simulink model "uas_sim"  (R2020b)
settings: Solver=VariableStepAuto  StartTime=0.0  StopTime=10.0  RelTol=1e-3  SampleTimeConstraint=STIndependent
undefined symbols (not defined in the file): Aircraft, datetime, datevec, Earth, Env, InitCond, WGS84
libraries: aerolibconvert2 x8, simulink x8, aerolibadyn x3, aerolibasang x3, aerolibtransform2 x2, aerolibatmos2 x1, sharedutil x1, aerolibbdyn x1, shared6dof x1, aerolibgravity2 x1
(part 1 of 2)
settings Model: Creator=brian  LastModifiedBy=brian

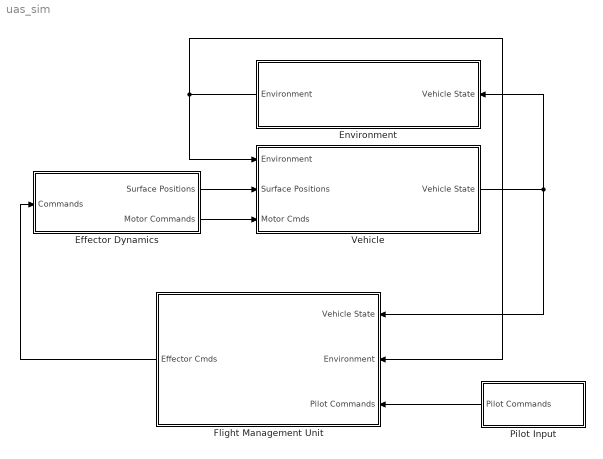
== system uas_sim ==
  Effector Dynamics : Subsystem
      settings: PortSchema="{\"entries\":[{\"content\":{\"sides\":[{\"content\":{\"connectorIds\":[]},\"type\":\"ConnectorPlacement.EquallySpacedRectSide\",\"uuid\":\"b20f7590-d69b-48b8-beb1-2fb7d3ab0357\"},{\"content\":{\"connectorIds\":[],\"side\":\"RIGHT\"},\"type\":\"ConnectorPlacement.EquallySpacedRectSide\",\"uuid\":\"07801f8a-7756-483e-a050-3c2fccc33404\"},{\"content\":{\"connectorIds\":[\"Out1\",\"Out2\"],\"side\":\"TOP\"},\"type\":\"ConnectorPlacement.EquallySpacedRectSide\",\"uuid\":\"ce3c3c94-ed36-4103-b079-69dcaeaf21e9\"},{\"content\":{\"connectorIds\":[\"In1\"],\"side\":\"BOTTOM\"},\"type\":\"ConnectorPlacement.EquallySpacedRectSide\",\"uuid\":\"ba78b819-a471-4bc3-b479-e6a973cfe14f\"},{\"content\":{\"connectorIds\":[],\"side\":\"HIDDEN\"},\"type\":\"ConnectorPlacement.EquallySpacedRectSide\",\"uuid\":\"3cf915a5-25a1-4380-9090-9561533312da\"}]},\"type\":\"ConnectorPlacement.EquallySpacedConnector\",\"uuid\":\"7ef4ddaa-ccd2-4778-89ce-8b4685524e82\"}],\"packageUris\":[\"http://schema.mathworks.com/mf0/Connector/R2020b\"],\"version\":\"1.0\"}"
  Environment : Subsystem
  Flight Management Unit : Subsystem
  Pilot Input : Subsystem
  Vehicle : Subsystem
  wires:
  Vehicle/1(Vehicle State) -> Environment/1(Vehicle State), Flight Management Unit/1(Vehicle State)
  Pilot Input/1(Pilot Commands) -> Flight Management Unit/3(Pilot Commands)
  Environment/1(Environment) -> Vehicle/1(Environment), Flight Management Unit/2(Environment)
  Flight Management Unit/1(Effector Cmds) -> Effector Dynamics/1(Commands)
  Effector Dynamics/1(Surface Positions) -> Vehicle/2(Surface Positions)
  Effector Dynamics/2(Motor Commands) -> Vehicle/3(Motor Cmds)

== system uas_sim/Effector Dynamics ==
  Commands : Inport
  Actuator Dynamics : Subsystem
  Bus Selector : BusSelector  OutputSignals=PWM,SBUS
  Mux : Mux  Inputs=2
  Selector : Selector  InputPortWidth=Aircraft.Eff.nCh  IndexOptions=Index vector (dialog)  Indices=Aircraft.Surf.map  OutputSizes=1
  Selector1 : Selector  InputPortWidth=Aircraft.Eff.nCh  IndexOptions=Index vector (dialog)  Indices=Aircraft.Motor.map  OutputSizes=1
  Surface Positions : Outport
  Motor Commands : Outport  Port=2
  wires:
  Commands/1 -> Bus Selector/1
  Bus Selector/1 -> Mux/1  "<PWM>"
  Bus Selector/2 -> Mux/2  "<SBUS>"
  Mux/1 -> Selector1/1, Selector/1
  Actuator Dynamics/1(Position) -> Surface Positions/1
  Selector/1 -> Actuator Dynamics/1(Command)
  Selector1/1 -> Motor Commands/1

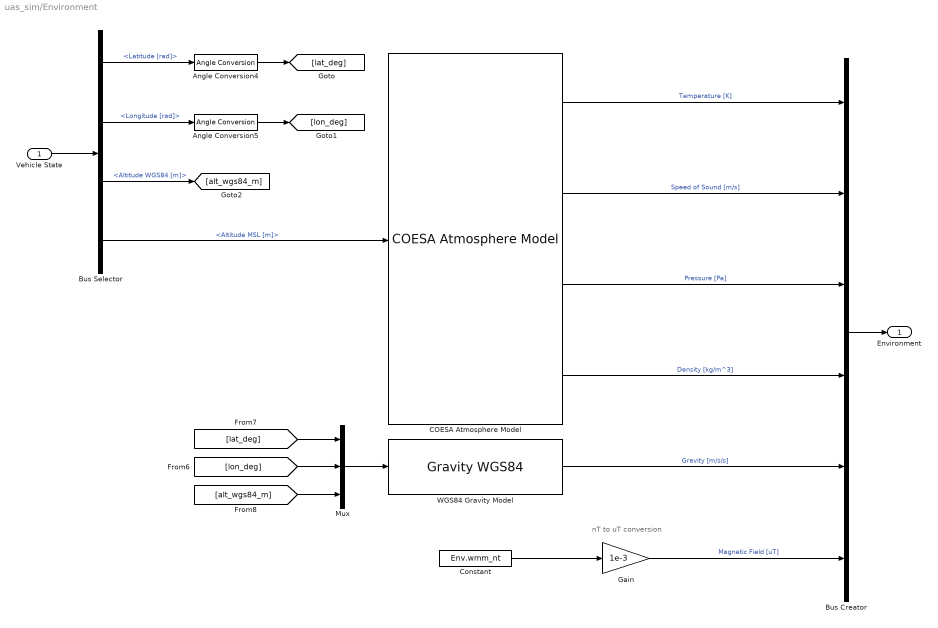
== system uas_sim/Environment ==
  note: nT to uT conversion
  Vehicle State : Inport
  Angle Conversion4 : aerolibconvert2/Angle Conversion  IU=rad  OU=deg
  Angle Conversion5 : aerolibconvert2/Angle Conversion  IU=rad  OU=deg
  Bus Creator : BusCreator  Inputs=6
  Bus Selector : BusSelector  OutputSignals=Latitude [rad],Longitude [rad],Altitude WGS84 [m],Altitude MSL [m]
  COESA Atmosphere Model : aerolibatmos2/COESA Atmosphere Model  units=Metric (MKS)  spec=1976 COESA-extended U.S. Standard Atmosphere  model=Profile  profile_var=High temperature  profile_percent=1%  profile_alt=5 km (16404 ft)  envelope_var=High temperature  envelope_percent=1%  action=Warning
  Constant : Constant  Value=Env.wmm_nt
  Gain : Gain  Gain=1e-3
  Mux : Mux  Inputs=3
  "WGS84 Gravity Model  " : GravityWGS84
  Environment : Outport
  wires:
  [lon_deg] -> Mux/2
  COESA Atmosphere Model/4 -> Bus Creator/4  "Density [kg/m^3]"
  Mux/1 -> "WGS84 Gravity Model  "/1
  Bus Selector/3 -> [alt_wgs84_m]  "<Altitude WGS84 [m]>"
  Vehicle State/1 -> Bus Selector/1
  Bus Selector/2 -> Angle Conversion5/1  "<Longitude [rad]>"
  COESA Atmosphere Model/2 -> Bus Creator/2  "Speed of Sound [m/s]"
  Bus Selector/4 -> COESA Atmosphere Model/1  "<Altitude MSL [m]>"
  [alt_wgs84_m] -> Mux/3
  Angle Conversion4/1 -> [lat_deg]
  [lat_deg] -> Mux/1
  Bus Creator/1 -> Environment/1
  Constant/1 -> Gain/1
  Gain/1 -> Bus Creator/6  "Magnetic Field [uT]"
  "WGS84 Gravity Model  "/1 -> Bus Creator/5  "Gravity [m/s/s]"
  Bus Selector/1 -> Angle Conversion4/1  "<Latitude [rad]>"
  COESA Atmosphere Model/3 -> Bus Creator/3  "Pressure [Pa]"
  COESA Atmosphere Model/1 -> Bus Creator/1  "Temperature [K]"
  Angle Conversion5/1 -> [lon_deg]

== system uas_sim/Flight Management Unit ==
  Vehicle State : Inport
  Environment : Inport  Port=2
  Pilot Commands : Inport  Port=3
  SenProc Model : Subsystem
      settings: PortSchema="{\"entries\":[{\"content\":{\"sides\":[{\"content\":{\"connectorIds\":[]},\"type\":\"ConnectorPlacement.EquallySpacedRectSide\",\"uuid\":\"b20f7590-d69b-48b8-beb1-2fb7d3ab0357\"},{\"content\":{\"connectorIds\":[],\"side\":\"RIGHT\"},\"type\":\"ConnectorPlacement.EquallySpacedRectSide\",\"uuid\":\"07801f8a-7756-483e-a050-3c2fccc33404\"},{\"content\":{\"connectorIds\":[\"In1\",\"In2\"],\"side\":\"TOP\"},\"type\":\"ConnectorPlacement.EquallySpacedRectSide\",\"uuid\":\"ce3c3c94-ed36-4103-b079-69dcaeaf21e9\"},{\"content\":{\"connectorIds\":[\"Out1\"],\"side\":\"BOTTOM\"},\"type\":\"ConnectorPlacement.EquallySpacedRectSide\",\"uuid\":\"ba78b819-a471-4bc3-b479-e6a973cfe14f\"},{\"content\":{\"connectorIds\":[],\"side\":\"HIDDEN\"},\"type\":\"ConnectorPlacement.EquallySpacedRectSide\",\"uuid\":\"3cf915a5-25a1-4380-9090-9561533312da\"}]},\"type\":\"ConnectorPlacement.EquallySpacedConnector\",\"uuid\":\"7ef4ddaa-ccd2-4778-89ce-8b4685524e82\"}],\"packageUris\":[\"http://schema.mathworks.com/mf0/Connector/R2020b\"],\"version\":\"1.0\"}"
  Sensor Models : Subsystem
      settings: PortSchema="{\"entries\":[{\"content\":{\"sides\":[{\"content\":{\"connectorIds\":[]},\"type\":\"ConnectorPlacement.EquallySpacedRectSide\",\"uuid\":\"b20f7590-d69b-48b8-beb1-2fb7d3ab0357\"},{\"content\":{\"connectorIds\":[],\"side\":\"RIGHT\"},\"type\":\"ConnectorPlacement.EquallySpacedRectSide\",\"uuid\":\"07801f8a-7756-483e-a050-3c2fccc33404\"},{\"content\":{\"connectorIds\":[\"In1\",\"In2\"],\"side\":\"TOP\"},\"type\":\"ConnectorPlacement.EquallySpacedRectSide\",\"uuid\":\"ce3c3c94-ed36-4103-b079-69dcaeaf21e9\"},{\"content\":{\"connectorIds\":[\"Out1\"],\"side\":\"BOTTOM\"},\"type\":\"ConnectorPlacement.EquallySpacedRectSide\",\"uuid\":\"ba78b819-a471-4bc3-b479-e6a973cfe14f\"},{\"content\":{\"connectorIds\":[],\"side\":\"HIDDEN\"},\"type\":\"ConnectorPlacement.EquallySpacedRectSide\",\"uuid\":\"3cf915a5-25a1-4380-9090-9561533312da\"}]},\"type\":\"ConnectorPlacement.EquallySpacedConnector\",\"uuid\":\"7ef4ddaa-ccd2-4778-89ce-8b4685524e82\"}],\"packageUris\":[\"http://schema.mathworks.com/mf0/Connector/R2020b\"],\"version\":\"1.0\"}"
  Vehicle Management System : Subsystem  TreatAsAtomicUnit=on
  Effector Cmds : Outport
  wires:
  Pilot Commands/1 -> Vehicle Management System/3(Inceptor Data)
  Vehicle Management System/1(Effector Cmds) -> Effector Cmds/1
  Environment/1 -> SenProc Model/1(Environment), Sensor Models/1(Environment)
  Vehicle State/1 -> SenProc Model/2(Vehicle State), Sensor Models/2(Vehicle State)
  Sensor Models/1(Sensors) -> Vehicle Management System/1(Sensor Data)
  SenProc Model/1(SenProc Data) -> Vehicle Management System/2(SenProc Data)

== system uas_sim/Pilot Input ==
  note: - Throttle is a 0 - 1 input
      | - Pitch, roll, and yaw are +/- 1 inputs
      | - Mode 0, 1, and 2 are mode switchs tied to 3 position switches on the pilot transmitter, each sending a value of 0, 1, or 2 corresponding to the switch position
      | - Throttle enable is a motor safety switch, 0 indicates that the motor should be safed (i.e. sent an idle command) and a value of 1 means that the motor can be used.
  Bus Creator : BusCreator  Inputs=8
  Constant : Constant  Value=0  OutDataTypeStr=int8
  Constant1 : Constant  Value=0  OutDataTypeStr=int8
  Constant2 : Constant  Value=0  OutDataTypeStr=int8
  Constant3 : Constant  Value=0  OutDataTypeStr=boolean
  Constant{4..7} (4 alike) : Constant  Value=0  OutDataTypeStr=single
  Pilot Commands : Outport
  wires:
  Bus Creator/1 -> Pilot Commands/1
  Constant/1 -> Bus Creator/5  "Mode 0"
  Constant1/1 -> Bus Creator/6  "Mode 1"
  Constant2/1 -> Bus Creator/7  "Mode 2"
  Constant3/1 -> Bus Creator/8  "Throttle Enable"
  Constant4/1 -> Bus Creator/1  "Throttle"
  Constant5/1 -> Bus Creator/2  "Pitch"
  Constant6/1 -> Bus Creator/3  "Roll"
  Constant7/1 -> Bus Creator/4  "Yaw"

== system uas_sim/Vehicle ==
  Environment : Inport
  Surface Positions : Inport  Port=2  PortDimensions=Aircraft.Surf.nSurf
  Motor Cmds : Inport  Port=3
  Bus Creator : BusCreator  Inputs=25
  Bus Selector : BusSelector  OutputSignals=Gravity [m/s/s],Density [kg/m^3],Speed of Sound [m/s]
  Bus Selector1 : BusSelector  OutputSignals=Body Velocity [m/s],Body Rotational Rate [rad/s],Dynamic Pressure [Pa],Airspeed [m/s],Angle of Attack [rad],Sideslip Angle [rad],DCM_be
  Forces and Moments : Subsystem
  Vehicle Model : Subsystem
  Vehicle State : Outport
  wires:
  Bus Selector/1 -> Forces and Moments/10(Gravity [m/s/s])  "<Gravity [m/s/s]>"
  Bus Selector1/1 -> Forces and Moments/1(Body Velocity [m/s])  "<Body Velocity [m/s]>"
  Bus Selector1/2 -> Forces and Moments/2(Body Rotational Rate [rad/s])  "<Body Rotational Rate [rad/s]>"
  Vehicle Model/20(Angle of Attack Rate [rad/s]) -> Bus Creator/20  "Angle of Attack Rate [rad/s]"
  Bus Selector1/4 -> Forces and Moments/4(Airspeed [m/s])  "<Airspeed [m/s]>"
  Bus Selector1/6 -> Forces and Moments/6(Sideslip Angle [rad])  "<Sideslip Angle [rad]>"
  Bus Selector1/3 -> Forces and Moments/3(Dynamic Pressure [Pa])  "<Dynamic Pressure [Pa]>"
  Vehicle Model/4(Altitude MSL [m]) -> Bus Creator/4  "Altitude MSL [m]"
  Vehicle Model/25(DCM_be) -> Bus Creator/25  "DCM_be"
  Vehicle Model/16(Dynamic Pressure [Pa]) -> Bus Creator/16  "Dynamic Pressure [Pa]"
  Vehicle Model/22(Sideslip Angle Rate [rad/s]) -> Bus Creator/22  "Sideslip Angle Rate [rad/s]"
  Vehicle Model/21(Sideslip Angle [rad]) -> Bus Creator/21  "Sideslip Angle [rad]"
  Vehicle Model/24(Flight Path Angle [rad]) -> Bus Creator/24  "Flight Path Angle [rad]"
  Vehicle Model/11(Yaw [rad]) -> Bus Creator/11  "Yaw [rad]"
  Vehicle Model/18(Mach) -> Bus Creator/18  "Mach"
  Vehicle Model/5(Altitude AGL [m]) -> Bus Creator/5  "Altitude AGL [m]"
  Bus Selector1/7 -> Forces and Moments/7(DCM_be)  "<DCM_be>"
  Bus Selector1/5 -> Forces and Moments/5(Angle of Attack [rad])  "<Angle of Attack [rad]>"
  Bus Selector/2 -> Forces and Moments/11(Density [kg/m^3]), Vehicle Model/3(Density [kg/m^3])  "<Density [kg/m^3]>"
  Vehicle Model/6(NED Position [m]) -> Bus Creator/6  "NED Position [m]"
  Vehicle Model/23(Ground Track [rad]) -> Bus Creator/23  "Ground Track [rad]"
  Vehicle Model/10(Roll [rad]) -> Bus Creator/10  "Roll [rad]"
  Vehicle Model/7(NED Velocity [m/s]) -> Bus Creator/7  "NED Velocity [m/s]"
  Surface Positions/1 -> Forces and Moments/8(Surface Positions [rad])
  Vehicle Model/17(Airspeed [m/s]) -> Bus Creator/17  "Airspeed [m/s]"
  Vehicle Model/15(Body Rotational Accel [rad/s/s]) -> Bus Creator/15  "Body Rotational Accel [rad/s/s]"
  Vehicle Model/14(Body Rotational Rate [rad/s]) -> Bus Creator/14  "Body Rotational Rate [rad/s]"
  Vehicle Model/13(Body Accel [m/s/s]) -> Bus Creator/13  "Body Accel [m/s/s]"
  Vehicle Model/9(Pitch [rad]) -> Bus Creator/9  "Pitch [rad]"
  Vehicle Model/8(NED Accel [m/s/s]) -> Bus Creator/8  "NED Accel [m/s/s]"
  Forces and Moments/2(Mxyz [N-m]) -> Vehicle Model/2(Mxyz [N-m])
  Environment/1 -> Bus Selector/1
  Bus Selector/3 -> Vehicle Model/4(Speed of Sound [m/s])  "<Speed of Sound [m/s]>"
  Bus Creator/1 -> Bus Selector1/1, Vehicle State/1
  Forces and Moments/1(Fxyz [N]) -> Vehicle Model/1(Fxyz [N])
  Vehicle Model/19(Angle of Attack [rad]) -> Bus Creator/19  "Angle of Attack [rad]"
  Vehicle Model/3(Altitude WGS84 [m]) -> Bus Creator/3  "Altitude WGS84 [m]"
  Motor Cmds/1 -> Forces and Moments/9(Motor Cmds)
  Vehicle Model/2(Longitude [rad]) -> Bus Creator/2  "Longitude [rad]"
  Vehicle Model/1(Latitude [rad]) -> Bus Creator/1  "Latitude [rad]"
  Vehicle Model/12(Body Velocity [m/s]) -> Bus Creator/12  "Body Velocity [m/s]"

== system uas_sim/Effector Dynamics/Actuator Dynamics ==
  Command : Inport
  Integrator : Integrator  InitialCondition=InitCond.surf_rad  LimitOutput=on  UpperSaturationLimit=Aircraft.Surf.Limit.pos_deg  LowerSaturationLimit=Aircraft.Surf.Limit.neg_deg
  Saturation : Saturate  UpperLimit=Aircraft.Surf.Limit.rate_dps  LowerLimit=-Aircraft.Surf.Limit.rate_dps
  Sum : Sum  Inputs=-+|
  Position : Outport
  wires:
  Command/1 -> Sum/2
  Saturation/1 -> Integrator/1
  Integrator/1 -> Position/1, Sum/1
  Sum/1 -> Saturation/1

== system uas_sim/Flight Management Unit/SenProc Model ==
  Environment : Inport
  Vehicle State : Inport  Port=2
  Air Data : Subsystem
  Bus Creator : BusCreator  Inputs=2
  Bus Selector : BusSelector  OutputSignals=Pressure [Pa]
  Bus Selector1 : BusSelector  OutputSignals=Dynamic Pressure [Pa],Body Accel [m/s/s],Body Rotational Rate [rad/s],Pitch [rad],Roll [rad],Yaw [rad],Latitude [rad],Longitude [rad],Altitude WGS84 [m],NED Velocity [m/s]
  INS / EKF : Subsystem
  SenProc Data : Outport
  wires:
  Environment/1 -> Bus Selector/1
  Bus Selector/1 -> Air Data/1(Static Pressure [Pa])  "<Pressure [Pa]>"
  Air Data/1(Airdata) -> Bus Creator/1  "Airdata"
  INS / EKF/1(INS) -> Bus Creator/2  "INS"
  Bus Creator/1 -> SenProc Data/1
  Vehicle State/1 -> Bus Selector1/1
  Bus Selector1/10 -> INS / EKF/9(NED Velocity [m/s])  "<NED Velocity [m/s]>"
  Bus Selector1/9 -> INS / EKF/8(Altitude WGS84 [m])  "<Altitude WGS84 [m]>"
  Bus Selector1/8 -> INS / EKF/7(Longitude [rad])  "<Longitude [rad]>"
  Bus Selector1/7 -> INS / EKF/6(Latitude [rad])  "<Latitude [rad]>"
  Bus Selector1/6 -> INS / EKF/5(Yaw [rad])  "<Yaw [rad]>"
  Bus Selector1/5 -> INS / EKF/4(Roll [rad])  "<Roll [rad]>"
  Bus Selector1/4 -> INS / EKF/3(Pitch [rad])  "<Pitch [rad]>"
  Bus Selector1/3 -> INS / EKF/2(Gyro [rad/s])  "<Body Rotational Rate [rad/s]>"
  Bus Selector1/2 -> INS / EKF/1(Accel [m/s/s])  "<Body Accel [m/s/s]>"
  Bus Selector1/1 -> Air Data/2(Differential Pressure [Pa])  "<Dynamic Pressure [Pa]>"

== system uas_sim/Flight Management Unit/Sensor Models ==
  Environment : Inport
  Vehicle State : Inport  Port=2
  Airdata : Subsystem
  Bus Creator : BusCreator  Inputs=4
  Bus Selector : BusSelector  OutputSignals=Body Rotational Rate [rad/s],Body Accel [m/s/s],DCM_be
  Bus Selector1 : BusSelector  OutputSignals=Latitude [rad],Longitude [rad],Altitude WGS84 [m],NED Velocity [m/s]
  Bus Selector2 : BusSelector  OutputSignals=Dynamic Pressure [Pa]
  Bus Selector3 : BusSelector  OutputSignals=Gravity [m/s/s],Magnetic Field [uT]
  Bus Selector4 : BusSelector  OutputSignals=Pressure [Pa]
  Clock : Clock
      settings: Decimation=1e6
  GNSS : Subsystem
  IMU : Subsystem
  Sensors : Outport
  wires:
  Bus Creator/1 -> Sensors/1
  Clock/1 -> Bus Creator/1  "System Time [s]"
  IMU/1(IMU Data) -> Bus Creator/2  "IMU"
  GNSS/1(GNSS Data) -> Bus Creator/3  "GNSS"
  Airdata/1(Airdata) -> Bus Creator/4  "Airdata"
  Vehicle State/1 -> Bus Selector2/1, Bus Selector1/1, Bus Selector/1
  Bus Selector/1 -> IMU/1(Body Rotational Rate [rad/s])  "<Body Rotational Rate [rad/s]>"
  Bus Selector/2 -> IMU/2(Body Accel [m/s/s])  "<Body Accel [m/s/s]>"
  Bus Selector/3 -> IMU/3(DCM_be)  "<DCM_be>"
  Bus Selector1/1 -> GNSS/1(Latitude [rad])  "<Latitude [rad]>"
  Bus Selector1/2 -> GNSS/2("Longitude [rad] ")  "<Longitude [rad]>"
  Bus Selector1/3 -> GNSS/3(Altitude WGS84 [m])  "<Altitude WGS84 [m]>"
  Bus Selector1/4 -> GNSS/4(NED Velocity [m/s])  "<NED Velocity [m/s]>"
  Bus Selector2/1 -> Airdata/1(Dynamic Pressure [Pa])  "<Dynamic Pressure [Pa]>"
  Environment/1 -> Bus Selector4/1, Bus Selector3/1
  Bus Selector3/1 -> IMU/4(Gravity [m/s/s])  "<Gravity [m/s/s]>"
  Bus Selector3/2 -> IMU/5(Magnetic Field [uT])  "<Magnetic Field [uT]>"
  Bus Selector4/1 -> Airdata/2(Static Pressure [Pa])  "<Pressure [Pa]>"

== system uas_sim/Flight Management Unit/Vehicle Management System ==
  Sensor Data : Inport
  SenProc Data : Inport  Port=2
  Inceptor Data : Inport  Port=3
  Effector Cmd Mapping : Subsystem
  Inceptor Data Mapping : Subsystem
  SenProc Data Mapping : Subsystem
  Sensor Data Mapping : Subsystem
  Terminator : Terminator
  Unit Delay : UnitDelay  SampleTime=-1  HasFrameUpgradeWarning=on
  Unit Delay1 : UnitDelay  SampleTime=-1  HasFrameUpgradeWarning=on
  Unit Delay2 : UnitDelay  SampleTime=-1  HasFrameUpgradeWarning=on
  VMS Autocode : ModelReference  ModelNameDialog=baseline.slx  SimulationMode=Normal  ModelReferenceVersion=1.47
  Effector Cmds : Outport
  wires:
  Unit Delay1/1 -> VMS Autocode/1
  Sensor Data Mapping/1(Non-virtual) -> Unit Delay1/1
  Inceptor Data/1 -> Inceptor Data Mapping/1(Virtual)
  Inceptor Data Mapping/1(Non-virtual) -> Unit Delay/1
  Sensor Data/1 -> Sensor Data Mapping/1(Virtual)
  VMS Autocode/2 -> Effector Cmd Mapping/1(Non-virtual)
  Effector Cmd Mapping/1(Virtual) -> Effector Cmds/1
  Unit Delay/1 -> VMS Autocode/3
  VMS Autocode/1 -> Terminator/1
  SenProc Data Mapping/1(Non-virtual) -> Unit Delay2/1
  SenProc Data/1 -> SenProc Data Mapping/1(Virtual)
  Unit Delay2/1 -> VMS Autocode/2

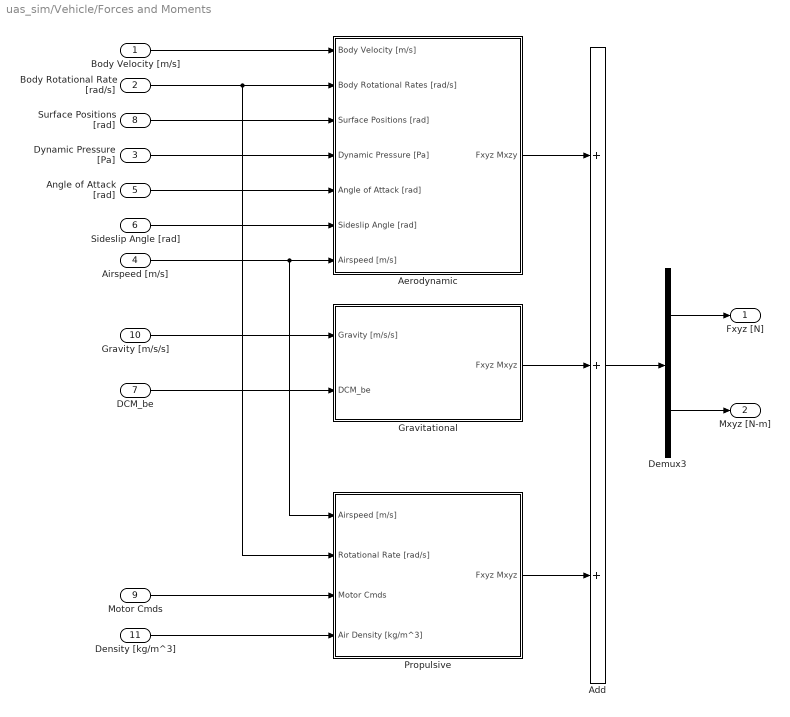
== system uas_sim/Vehicle/Forces and Moments ==
  Body Velocity [m/s] : Inport
  Body Rotational Rate [rad/s] : Inport  Port=2
  Dynamic Pressure [Pa] : Inport  Port=3
  Airspeed [m/s] : Inport  Port=4
  Angle of Attack [rad] : Inport  Port=5
  Sideslip Angle [rad] : Inport  Port=6
  DCM_be : Inport  Port=7
  Surface Positions [rad] : Inport  Port=8
  Motor Cmds : Inport  Port=9
  Gravity [m/s/s] : Inport  Port=10
  Density [kg/m^3] : Inport  Port=11
  Add : Sum  Inputs=+++
  Aerodynamic : Subsystem
  Demux3 : Demux  Outputs=2
  Gravitational : Subsystem
  Propulsive : Subsystem
  Fxyz [N] : Outport
  Mxyz [N-m] : Outport  Port=2
  wires:
  Surface Positions [rad]/1 -> Aerodynamic/3(Surface Positions [rad])
  Add/1 -> Demux3/1
  Gravity [m/s/s]/1 -> Gravitational/1(Gravity [m/s/s])
  Motor Cmds/1 -> Propulsive/3(Motor Cmds)
  Demux3/1 -> Fxyz [N]/1
  Sideslip Angle [rad]/1 -> Aerodynamic/6(Sideslip Angle [rad])
  Dynamic Pressure [Pa]/1 -> Aerodynamic/4(Dynamic Pressure [Pa])
  DCM_be/1 -> Gravitational/2(DCM_be)
  Angle of Attack [rad]/1 -> Aerodynamic/5(Angle of Attack [rad])
  Propulsive/1(Fxyz Mxyz) -> Add/3
  Body Rotational Rate [rad/s]/1 -> Propulsive/2(Rotational Rate [rad/s]), Aerodynamic/2(Body Rotational Rates [rad/s])
  Demux3/2 -> Mxyz [N-m]/1
  Airspeed [m/s]/1 -> Propulsive/1(Airspeed [m/s]), Aerodynamic/7(Airspeed [m/s])
  Aerodynamic/1(Fxyz Mxzy) -> Add/1
  Body Velocity [m/s]/1 -> Aerodynamic/1(Body Velocity [m/s])
  Gravitational/1(Fxyz Mxyz) -> Add/2
  Density [kg/m^3]/1 -> Propulsive/4(Air Density [kg/m^3])

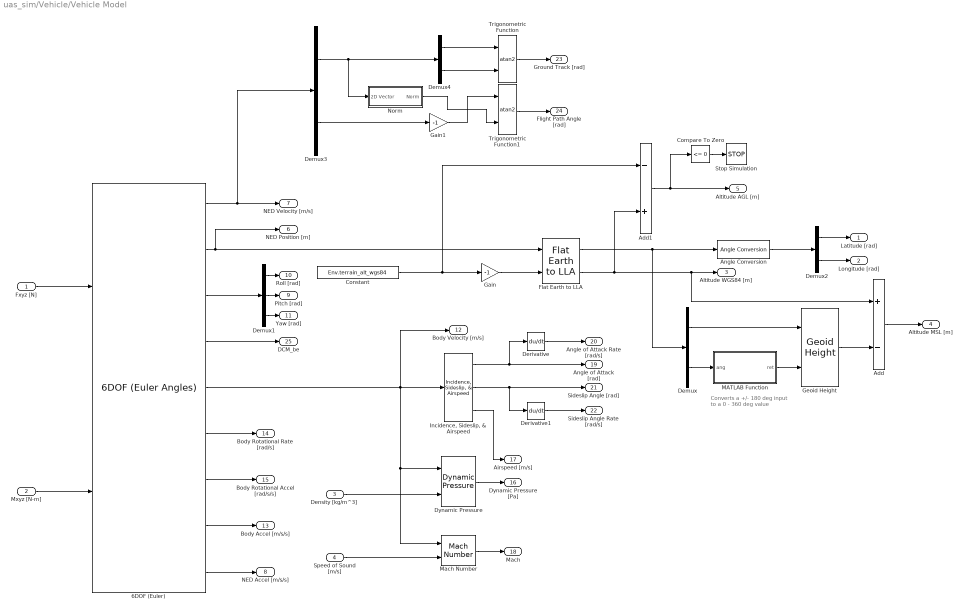
== system uas_sim/Vehicle/Vehicle Model ==
  note: Converts a +/- 180 deg
      | input to a 0 - 360 deg value
  Fxyz [N] : Inport
  Mxyz [N-m] : Inport  Port=2
  Density [kg/m^3] : Inport  Port=3
  Speed of Sound [m/s] : Inport  Port=4
  6DOF (Euler) : shared6dof/6DOF (Euler Angles)  units=Metric (MKS)  mtype=Fixed  rep=Euler Angles  xme_0=InitCond.ned_pos_m  Vm_0=InitCond.body_vel_mps  eul_0=InitCond.euler_rad  pm_0=InitCond.body_rot_rate_radps  mass_0=Aircraft.Mass.mass_kg  mass_e=0.5  mass_f=2.0  inertia=Aircraft.Mass.inertia_kgm2  inertia_e=eye(3)  inertia_f=2*eye(3)  k_quat=1.0  vre_flag=on  abi_flag=on  aMode=0  xme_statename=''  Vm_statename=''  eul_statename=''  quat_statename=''  pm_statename=''  mass_statename=''
      settings: SourceProductBaseCode=AE,PW,MT,UV,VE,VP
  Add : Sum  Inputs=+-
  Add1 : Sum  Inputs=-+
  Angle Conversion : aerolibconvert2/Angle Conversion  IU=deg  OU=rad
  Compare To Zero : simulink/Logic and Bit Operations/Compare To Zero  relop=<=  OutDataTypeStr=boolean
  Constant : Constant  Value=Env.terrain_alt_wgs84
  Demux : Demux  Outputs=2
  Demux1 : Demux  Outputs=3
  Demux2 : Demux  Outputs=2
  Demux3 : Demux  Outputs=[2 1]
  Demux4 : Demux  Outputs=2
  Derivative : Derivative
  Derivative1 : Derivative
  Dynamic Pressure : aerolibasang/Dynamic Pressure
  Flat Earth to LLA : aerolibtransform2/Flat Earth to LLA  units=Metric (MKS)  ptype=Earth (WGS84)  F=1/298.257223563  R=6378137  refPosPort=off  LL0=[rad2deg(InitCond.lat_rad) rad2deg(InitCond.lon_rad)]  psi=0
  Gain : Gain  Gain=-1
  Gain1 : Gain  Gain=-1
  Geoid Height : aerolibgravity2/Geoid Height  units=Metric (MKS)  gtype=EGM2008  datafile='geoidegm96grid'  dtype=double  action=Warning
      settings: SourceProductBaseCode=AE
  "Incidence, Sideslip, & Airspeed" : aerolibasang/Incidence, Sideslip, & Airspeed
  MATLAB Function : MATLAB Function  TreatAsAtomicUnit=on
  Mach Number : aerolibasang/Mach Number
      settings: SourceProductBaseCode=AE
  Norm : Subsystem
  Stop Simulation : Stop
  Trigonometric Function : Trigonometry  Operator=atan2
  Trigonometric Function1 : Trigonometry  Operator=atan2
  Latitude [rad] : Outport
  Longitude [rad] : Outport  Port=2
  Altitude WGS84 [m] : Outport  Port=3
  Altitude MSL [m] : Outport  Port=4
  Altitude AGL [m] : Outport  Port=5
  NED Position [m] : Outport  Port=6
  NED Velocity [m/s] : Outport  Port=7
  NED Accel [m/s/s] : Outport  Port=8
  Pitch [rad] : Outport  Port=9
  Roll [rad] : Outport  Port=10
  Yaw [rad] : Outport  Port=11
  Body Velocity [m/s] : Outport  Port=12
  Body Accel [m/s/s] : Outport  Port=13
  Body Rotational Rate [rad/s] : Outport  Port=14
  Body Rotational Accel [rad/s/s] : Outport  Port=15
  Dynamic Pressure [Pa] : Outport  Port=16
  Airspeed [m/s] : Outport  Port=17
  Mach : Outport  Port=18
  Angle of Attack [rad] : Outport  Port=19
  Angle of Attack Rate [rad/s] : Outport  Port=20
  Sideslip Angle [rad] : Outport  Port=21
  Sideslip Angle Rate [rad/s] : Outport  Port=22
  Ground Track [rad] : Outport  Port=23
  Flight Path Angle [rad] : Outport  Port=24
  DCM_be : Outport  Port=25
  wires:
  Fxyz [N]/1 -> 6DOF (Euler)/1
  Mxyz [N-m]/1 -> 6DOF (Euler)/2
  6DOF (Euler)/5 -> Body Velocity [m/s]/1, "Incidence, Sideslip, & Airspeed"/1, Dynamic Pressure/1, Mach Number/1
  Flat Earth to LLA/1 -> Demux/1, Angle Conversion/1
  Flat Earth to LLA/2 -> Add1/2, Add/1, Altitude WGS84 [m]/1
  Geoid Height/1 -> Add/2
  Demux/2 -> MATLAB Function/1(ang)
  Demux/1 -> Geoid Height/1
  "Incidence, Sideslip, & Airspeed"/3 -> Airspeed [m/s]/1
  Density [kg/m^3]/1 -> Dynamic Pressure/2
  Angle Conversion/1 -> Demux2/1
  6DOF (Euler)/4 -> DCM_be/1
  Demux1/1 -> Roll [rad]/1
  6DOF (Euler)/3 -> Demux1/1
  Demux1/2 -> Pitch [rad]/1
  Demux1/3 -> Yaw [rad]/1
  Dynamic Pressure/1 -> Dynamic Pressure [Pa]/1
  "Incidence, Sideslip, & Airspeed"/1 -> Derivative/1, Angle of Attack [rad]/1
  "Incidence, Sideslip, & Airspeed"/2 -> Derivative1/1, Sideslip Angle [rad]/1
  Add/1 -> Altitude MSL [m]/1
  Gain/1 -> Flat Earth to LLA/2
  Demux2/2 -> Longitude [rad]/1
  Demux2/1 -> Latitude [rad]/1
  6DOF (Euler)/2 -> NED Position [m]/1, Flat Earth to LLA/1
  6DOF (Euler)/6 -> Body Rotational Rate [rad/s]/1
  6DOF (Euler)/7 -> Body Rotational Accel [rad/s/s]/1
  6DOF (Euler)/8 -> Body Accel [m/s/s]/1
  6DOF (Euler)/1 -> Demux3/1, NED Velocity [m/s]/1
  MATLAB Function/1(ret) -> Geoid Height/2
  Demux3/1 -> Norm/1(2D Vector), Demux4/1
  Demux4/1 -> Trigonometric Function/1
  Demux4/2 -> Trigonometric Function/2
  Trigonometric Function/1 -> Ground Track [rad]/1
  Demux3/2 -> Gain1/1
  Gain1/1 -> Trigonometric Function1/1
  Norm/1(Norm) -> Trigonometric Function1/2
  Trigonometric Function1/1 -> Flight Path Angle [rad]/1
  6DOF (Euler)/9 -> NED Accel [m/s/s]/1
  Speed of Sound [m/s]/1 -> Mach Number/2
  Mach Number/1 -> Mach/1
  Derivative/1 -> Angle of Attack Rate [rad/s]/1
  Derivative1/1 -> Sideslip Angle Rate [rad/s]/1
  Constant/1 -> Add1/1, Gain/1
  Add1/1 -> Compare To Zero/1, Altitude AGL [m]/1
  Compare To Zero/1 -> Stop Simulation/1

== system uas_sim/Flight Management Unit/SenProc Model/Air Data ==
  Static Pressure [Pa] : Inport
  Differential Pressure [Pa] : Inport  Port=2
  Bus Creator : BusCreator  Inputs=4
  IAS : Subsystem
  Pressure Altitude : Subsystem
  Airdata : Outport
  wires:
  Bus Creator/1 -> Airdata/1
  IAS/1(IAS [m/s]) -> Bus Creator/3  "IAS [m/s]"
  Pressure Altitude/1(Pressure Altitude [m]) -> Bus Creator/2  "Pressure Altitude [m]"
  Static Pressure [Pa]/1 -> Bus Creator/1, Pressure Altitude/1(Static Pressure [Pa])  "Static Pressure"
  Differential Pressure [Pa]/1 -> Bus Creator/4, IAS/1(Differential Pressure [Pa])  "Differential Pressure [Pa]"

== system uas_sim/Flight Management Unit/SenProc Model/INS // EKF ==
  Accel [m/s/s] : Inport
  Gyro [rad/s] : Inport  Port=2
  Pitch [rad] : Inport  Port=3
  Roll [rad] : Inport  Port=4
  Yaw [rad] : Inport  Port=5
  Latitude [rad] : Inport  Port=6
  Longitude [rad] : Inport  Port=7
  Altitude WGS84 [m] : Inport  Port=8
  NED Velocity [m/s] : Inport  Port=9
  Bus Creator : BusCreator  Inputs=9
  INS : Outport
  wires:
  Bus Creator/1 -> INS/1
  Accel [m/s/s]/1 -> Bus Creator/1  "Accel [m/s/s]"
  Gyro [rad/s]/1 -> Bus Creator/2  "Gyro [rad/s]"
  Pitch [rad]/1 -> Bus Creator/3  "Pitch [rad]"
  Roll [rad]/1 -> Bus Creator/4  "Roll [rad]"
  Yaw [rad]/1 -> Bus Creator/5  "Yaw [rad]"
  Latitude [rad]/1 -> Bus Creator/6  "Latitude [rad]"
  Longitude [rad]/1 -> Bus Creator/7  "Longitude [rad]"
  Altitude WGS84 [m]/1 -> Bus Creator/8  "Altitude WGS84 [m]"
  NED Velocity [m/s]/1 -> Bus Creator/9  "NED Velocity [m/s]"

== system uas_sim/Flight Management Unit/Sensor Models/Airdata ==
  Dynamic Pressure [Pa] : Inport
  Static Pressure [Pa] : Inport  Port=2
  Bus Creator : BusCreator  Inputs=2
  Differential Pressure Sensor : Subsystem
  Static Pressure Sensor : Subsystem
  Airdata : Outport
  wires:
  Dynamic Pressure [Pa]/1 -> Differential Pressure Sensor/1(Pressure)
  Differential Pressure Sensor/1(Sensed Value) -> Bus Creator/1  "Differential Pressure [Pa]"
  Bus Creator/1 -> Airdata/1
  Static Pressure Sensor/1(Sensed Value) -> Bus Creator/2  "Static Pressure [Pa]"
  Static Pressure [Pa]/1 -> Static Pressure Sensor/1(Pressure)

== system uas_sim/Flight Management Unit/Sensor Models/GNSS ==
  note: Simulates the lower sampling rate of GNSS receivers
  Latitude [rad] : Inport
  "Longitude [rad] " : Inport  Port=2
  Altitude WGS84 [m] : Inport  Port=3
  NED Velocity [m/s] : Inport  Port=4
  Band-Limited White Noise : simulink/Sources/Band-Limited White Noise  Cov=[Aircraft.Sensors.Gnss.horz_accuracy_m Aircraft.Sensors.Gnss.horz_accuracy_m Aircraft.Sensors.Gnss.vert_accuracy_m]  Ts=0.1  seed=[23341]
  Band-Limited White Noise2 : simulink/Sources/Band-Limited White Noise  Cov=Aircraft.Sensors.Gnss.vel_accuracy_mps * ones(3, 1)  Ts=0.1  seed=[23341]
  Bus Creator : BusCreator  Inputs=11
  Clock : Clock
  Pulse Generator : DiscretePulseGenerator  PulseType=Time based  Period=1/Aircraft.Sensors.Gnss.sample_rate_hz  PulseWidth=5
  Triggered Subsystem : Subsystem  TreatAsAtomicUnit=on
  GNSS Data : Outport
  wires:
  Bus Creator/1 -> GNSS Data/1
  Triggered Subsystem/5(Lat [rad]) -> Bus Creator/5  "Latitude [rad]"
  Triggered Subsystem/11(Velocity Accuracy [m/s]) -> Bus Creator/11  "Velocity Accuracy [m/s]"
  Triggered Subsystem/3(TOW [s]) -> Bus Creator/3  "TOW [s]"
  NED Velocity [m/s]/1 -> Triggered Subsystem/4(NED Velocity [m/s])
  Altitude WGS84 [m]/1 -> Triggered Subsystem/3(Altitude WGS84 [m])
  "Longitude [rad] "/1 -> Triggered Subsystem/2("Longitude [rad] ")
  Triggered Subsystem/9(Horizontal Accuracy [m]) -> Bus Creator/9  "Horizontal Accuracy [m]"
  Triggered Subsystem/10(Vertical Accuracy [m]) -> Bus Creator/10  "Vertical Accuracy [m]"
  Triggered Subsystem/4(Week) -> Bus Creator/4  "Week"
  Triggered Subsystem/1(Fix) -> Bus Creator/1  "Fix"
  Triggered Subsystem/7(Alt WGS84 [m]) -> Bus Creator/7  "Altitude WGS84 [m]"
  Clock/1 -> Triggered Subsystem/7(clock)
  Triggered Subsystem/6(Lon [rad]) -> Bus Creator/6  "Longitude [rad]"
  Triggered Subsystem/8(NED Vel [m/s]) -> Bus Creator/8  "NED Velocity [m/s]"
  Band-Limited White Noise/1 -> Triggered Subsystem/5(Position Noise [m])
  Triggered Subsystem/2(Num Satellites) -> Bus Creator/2  "Num Satellites"
  Pulse Generator/1 -> Triggered Subsystem/Trigger
  Band-Limited White Noise2/1 -> Triggered Subsystem/6(Velocity Noise [m/s])
  Latitude [rad]/1 -> Triggered Subsystem/1(Latitude [rad])

== system uas_sim/Flight Management Unit/Sensor Models/IMU ==
  Body Rotational Rate [rad/s] : Inport
  Body Accel [m/s/s] : Inport  Port=2
  DCM_be : Inport  Port=3
  Gravity [m/s/s] : Inport  Port=4
  Magnetic Field [uT] : Inport  Port=5
  Accelerometer : Subsystem
  Bus Creator : BusCreator  Inputs=3
  Gyro : Subsystem
  Magnetometer : Subsystem
  Product : Product  Multiplication=Matrix(*)
  Product1 : Product  Multiplication=Matrix(*)
  Reshape : Reshape  OutputDimensionality=Column vector (2-D)
  Reshape1 : Reshape
  Reshape2 : Reshape
  Reshape3 : Reshape  OutputDimensionality=Column vector (2-D)
  IMU Data : Outport
  wires:
  Body Accel [m/s/s]/1 -> Accelerometer/1(Body Accel [m/s/s]), Gyro/2(Body Accel [m/s/s])
  DCM_be/1 -> Product1/1, Product/1
  Gravity [m/s/s]/1 -> Reshape/1
  Bus Creator/1 -> IMU Data/1
  Reshape/1 -> Product/2
  Product/1 -> Reshape1/1
  Reshape1/1 -> Accelerometer/2(Gravitational Accel in Body Frame [m/s/s])
  Body Rotational Rate [rad/s]/1 -> Gyro/1(Body Rotational Rate [rad/s])
  Gyro/1(Gyro [rad/s]) -> Bus Creator/1  "Gyro [rad/s]"
  Accelerometer/1(Accelerometer [m/s/s]) -> Bus Creator/2  "Accelerometer [m/s/s]"
  Magnetometer/1(Magnetometer [uT]) -> Bus Creator/3  "Magnetometer [uT]"
  Reshape2/1 -> Magnetometer/1(Body Magnetic Field [uT])
  Product1/1 -> Reshape2/1
  Reshape3/1 -> Product1/2
  Magnetic Field [uT]/1 -> Reshape3/1

== system uas_sim/Flight Management Unit/Vehicle Management System/Effector Cmd Mapping ==
  Non-virtual : Inport
  Bus Creator : BusCreator  Inputs=2
  Bus Selector : BusSelector  OutputSignals=pwm,sbus
  Data Type Conversion : DataTypeConversion  OutDataTypeStr=double
  Data Type Conversion1 : DataTypeConversion  OutDataTypeStr=double
  Virtual : Outport
  wires:
  Non-virtual/1 -> Bus Selector/1
  Bus Selector/1 -> Data Type Conversion/1  "<pwm>"
  Bus Selector/2 -> Data Type Conversion1/1  "<sbus>"
  Data Type Conversion/1 -> Bus Creator/1  "PWM"
  Data Type Conversion1/1 -> Bus Creator/2  "SBUS"
  Bus Creator/1 -> Virtual/1

== system uas_sim/Flight Management Unit/Vehicle Management System/Inceptor Data Mapping ==
  Virtual : Inport
  Bus Creator : BusCreator  Inputs=8  OutDataTypeStr=Bus: InceptorData
      settings: InheritFromInputs=off
  Bus Selector : BusSelector  OutputSignals=Mode 0,Mode 1,Mode 2,Throttle Enable,Throttle,Pitch,Roll,Yaw
  Data Type Conversion : DataTypeConversion  OutDataTypeStr=int8
  Data Type Conversion1 : DataTypeConversion  OutDataTypeStr=int8
  Data Type Conversion2 : DataTypeConversion  OutDataTypeStr=int8
  Data Type Conversion3 : DataTypeConversion  OutDataTypeStr=boolean
  Data Type Conversion{4..7} (4 alike) : DataTypeConversion  OutDataTypeStr=single
  Non-virtual : Outport  OutDataTypeStr=Bus: InceptorData
  wires:
  Bus Selector/7 -> Data Type Conversion6/1  "<Roll>"
  Bus Selector/4 -> Data Type Conversion3/1  "<Throttle Enable>"
  Data Type Conversion3/1 -> Bus Creator/4  "throttle_en"
  Data Type Conversion/1 -> Bus Creator/1  "mode0"
  Bus Selector/1 -> Data Type Conversion/1  "<Mode 0>"
  Data Type Conversion1/1 -> Bus Creator/2  "mode1"
  Data Type Conversion2/1 -> Bus Creator/3  "mode2"
  Bus Selector/3 -> Data Type Conversion2/1  "<Mode 2>"
  Data Type Conversion5/1 -> Bus Creator/6  "pitch"
  Bus Selector/2 -> Data Type Conversion1/1  "<Mode 1>"
  Bus Selector/5 -> Data Type Conversion4/1  "<Throttle>"
  Data Type Conversion4/1 -> Bus Creator/5  "throttle"
  Bus Selector/6 -> Data Type Conversion5/1  "<Pitch>"
  Bus Selector/8 -> Data Type Conversion7/1  "<Yaw>"
  Data Type Conversion6/1 -> Bus Creator/7  "roll"
  Data Type Conversion7/1 -> Bus Creator/8  "yaw"
  Virtual/1 -> Bus Selector/1
  Bus Creator/1 -> Non-virtual/1

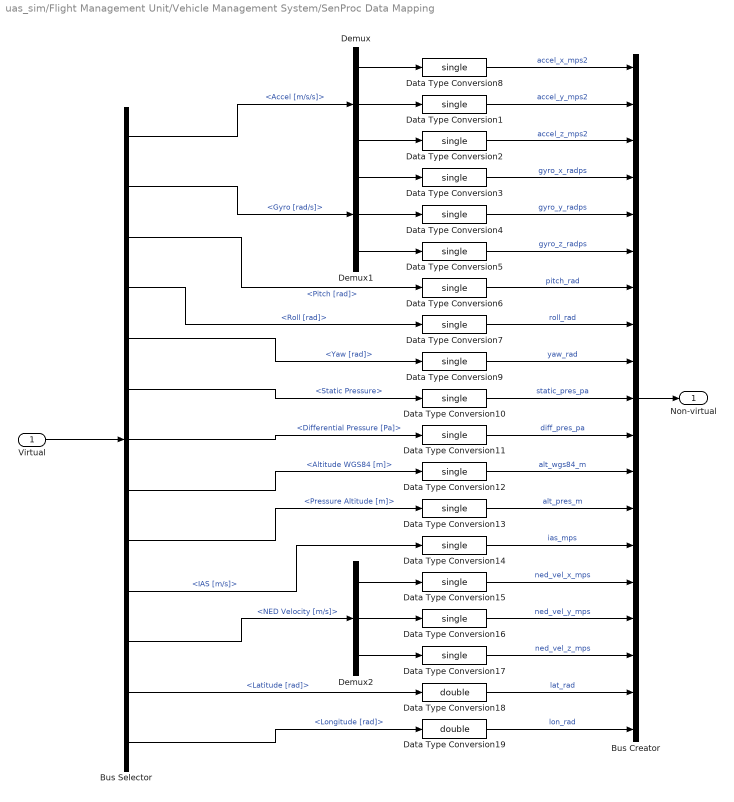
== system uas_sim/Flight Management Unit/Vehicle Management System/SenProc Data Mapping ==
  Virtual : Inport
  Bus Creator : BusCreator  Inputs=19  OutDataTypeStr=Bus: SenProcData
      settings: InheritFromInputs=off
  Bus Selector : BusSelector  OutputSignals=INS.Accel [m/s/s],INS.Gyro [rad/s],INS.Pitch [rad],INS.Roll [rad],INS.Yaw [rad],Airdata.Static Pressure,Airdata.Differential Pressure [Pa],INS.Altitude WGS84 [m],Airdata.Pressure Altitude [m],Airdata.IAS [m/s],INS.NED Velocity [m/s],INS.Latitude [rad],INS.Longitude [rad]
  Data Type Conversion{1..17} (17 alike) : DataTypeConversion  OutDataTypeStr=single
  Data Type Conversion18 : DataTypeConversion  OutDataTypeStr=double
  Data Type Conversion19 : DataTypeConversion  OutDataTypeStr=double
  Demux : Demux  Outputs=3
  Demux1 : Demux  Outputs=3
  Demux2 : Demux  Outputs=3
  Non-virtual : Outport  OutDataTypeStr=Bus: SenProcData
  wires:
  Virtual/1 -> Bus Selector/1
  Bus Creator/1 -> Non-virtual/1
  Bus Selector/1 -> Demux/1  "<Accel [m/s/s]>"
  Demux/1 -> Data Type Conversion8/1
  Demux/2 -> Data Type Conversion1/1
  Demux/3 -> Data Type Conversion2/1
  Data Type Conversion8/1 -> Bus Creator/1  "accel_x_mps2"
  Data Type Conversion1/1 -> Bus Creator/2  "accel_y_mps2"
  Data Type Conversion2/1 -> Bus Creator/3  "accel_z_mps2"
  Demux1/3 -> Data Type Conversion5/1
  Demux1/2 -> Data Type Conversion4/1
  Demux1/1 -> Data Type Conversion3/1
  Bus Selector/2 -> Demux1/1  "<Gyro [rad/s]>"
  Data Type Conversion3/1 -> Bus Creator/4  "gyro_x_radps"
  Data Type Conversion4/1 -> Bus Creator/5  "gyro_y_radps"
  Data Type Conversion5/1 -> Bus Creator/6  "gyro_z_radps"
  Data Type Conversion6/1 -> Bus Creator/7  "pitch_rad"
  Data Type Conversion7/1 -> Bus Creator/8  "roll_rad"
  Data Type Conversion9/1 -> Bus Creator/9  "yaw_rad"
  Bus Selector/3 -> Data Type Conversion6/1  "<Pitch [rad]>"
  Bus Selector/4 -> Data Type Conversion7/1  "<Roll [rad]>"
  Bus Selector/5 -> Data Type Conversion9/1  "<Yaw [rad]>"
  Bus Selector/6 -> Data Type Conversion10/1  "<Static Pressure>"
  Bus Selector/7 -> Data Type Conversion11/1  "<Differential Pressure [Pa]>"
  Bus Selector/8 -> Data Type Conversion12/1  "<Altitude WGS84 [m]>"
  Bus Selector/9 -> Data Type Conversion13/1  "<Pressure Altitude [m]>"
  Bus Selector/10 -> Data Type Conversion14/1  "<IAS [m/s]>"
  Data Type Conversion10/1 -> Bus Creator/10  "static_pres_pa"
  Data Type Conversion11/1 -> Bus Creator/11  "diff_pres_pa"
  Data Type Conversion12/1 -> Bus Creator/12  "alt_wgs84_m"
  Data Type Conversion13/1 -> Bus Creator/13  "alt_pres_m"
  Data Type Conversion14/1 -> Bus Creator/14  "ias_mps"
  Bus Selector/11 -> Demux2/1  "<NED Velocity [m/s]>"
  Bus Selector/13 -> Data Type Conversion19/1  "<Longitude [rad]>"
  Bus Selector/12 -> Data Type Conversion18/1  "<Latitude [rad]>"
  Data Type Conversion19/1 -> Bus Creator/19  "lon_rad"
  Data Type Conversion18/1 -> Bus Creator/18  "lat_rad"
  Demux2/1 -> Data Type Conversion15/1
  Demux2/2 -> Data Type Conversion16/1
  Demux2/3 -> Data Type Conversion17/1
  Data Type Conversion15/1 -> Bus Creator/15  "ned_vel_x_mps"
  Data Type Conversion16/1 -> Bus Creator/16  "ned_vel_y_mps"
  Data Type Conversion17/1 -> Bus Creator/17  "ned_vel_z_mps"

== system uas_sim/Flight Management Unit/Vehicle Management System/Sensor Data Mapping ==
  Virtual : Inport
  Air Data Mapping : Subsystem
  Bus Creator : BusCreator  Inputs=4  OutDataTypeStr=Bus: SensorData
      settings: InheritFromInputs=off
  Bus Selector : BusSelector  OutputSignals=System Time [s],IMU,GNSS,Airdata
  Data Type Conversion : DataTypeConversion  OutDataTypeStr=double
  GNSS Data Mapping : Subsystem
  IMU Data Mapping : Subsystem
  Non-virtual : Outport  OutDataTypeStr=Bus: SensorData
  wires:
  Bus Creator/1 -> Non-virtual/1
  Air Data Mapping/1(Non-virtual) -> Bus Creator/4  "airdata"
  GNSS Data Mapping/1(Non-virtual) -> Bus Creator/3  "gnss"
  IMU Data Mapping/1(Non-virtual) -> Bus Creator/2  "imu"
  Virtual/1 -> Bus Selector/1
  Bus Selector/4 -> Air Data Mapping/1(Virtual)  "<Airdata>"
  Bus Selector/3 -> GNSS Data Mapping/1(Virtual)  "<GNSS>"
  Bus Selector/2 -> IMU Data Mapping/1(Virtual)  "<IMU>"
  Bus Selector/1 -> Data Type Conversion/1  "<System Time [s]>"
  Data Type Conversion/1 -> Bus Creator/1  "sys_time_s"

== system uas_sim/Vehicle/Forces and Moments/Aerodynamic ==
  note: C6 = [CD, CY, CLift, CL, CM, CN]
  Body Velocity [m/s] : Inport
  Body Rotational Rates [rad/s] : Inport  Port=2
  Surface Positions [rad] : Inport  Port=3
  Dynamic Pressure [Pa] : Inport  Port=4
  Angle of Attack [rad] : Inport  Port=5
  Sideslip Angle [rad] : Inport  Port=6
  Airspeed [m/s] : Inport  Port=7
  Add : Sum  Inputs=+++
  Aerodynamic Forces and Moments Coef Axis Variant : Subsystem  Variant=on
  Base Airframe : Subsystem
  Control Derivatives : Subsystem
  Dynamic Derivatives : Subsystem
  Fxyz Mxzy : Outport
  wires:
  Base Airframe/1(C6) -> Add/1
  Dynamic Derivatives/1(dC6) -> Add/2
  Sideslip Angle [rad]/1 -> Base Airframe/2(Sideslip Angle [rad])
  Angle of Attack [rad]/1 -> Base Airframe/1(Angle of Attack [rad]), Control Derivatives/2(Angle of Attack [rad]), Dynamic Derivatives/3(Angle of Attack [rad])
  Body Rotational Rates [rad/s]/1 -> Dynamic Derivatives/2(Body Rotational Rate [rad/s])
  Airspeed [m/s]/1 -> Dynamic Derivatives/1(Airspeed [m/s])
  Surface Positions [rad]/1 -> Control Derivatives/1(Surface Positions [rad])
  Control Derivatives/1(dC6) -> Add/3
  Add/1 -> Aerodynamic Forces and Moments Coef Axis Variant/1(Coef)
  Body Velocity [m/s]/1 -> Aerodynamic Forces and Moments Coef Axis Variant/3(Body Velocity [m/s])
  Dynamic Pressure [Pa]/1 -> Aerodynamic Forces and Moments Coef Axis Variant/2(Dynamic Pressure [Pa])
  Aerodynamic Forces and Moments Coef Axis Variant/1(Fxyz Mxyz) -> Fxyz Mxzy/1

== system uas_sim/Vehicle/Forces and Moments/Gravitational ==
  Gravity [m/s/s] : Inport
  DCM_be : Inport  Port=2
  Gravity Moment : Constant  Value=[0 0 0]
  Mux : Mux  Inputs=2
  Product : Product
  Product1 : Product  Multiplication=Matrix(*)
  Reshape : Reshape  OutputDimensionality=Column vector (2-D)
  Reshape1 : Reshape
  UAV Mass : Constant  Value=Aircraft.Mass.mass_kg
  Fxyz Mxyz : Outport
  wires:
  UAV Mass/1 -> Product/2
  Product/1 -> Product1/2  "Gravity Force NED [N]"
  DCM_be/1 -> Product1/1
  Gravity Moment/1 -> Mux/2
  Mux/1 -> Fxyz Mxyz/1
  Reshape/1 -> Product/1
  Gravity [m/s/s]/1 -> Reshape/1
  Reshape1/1 -> Mux/1
  Product1/1 -> Reshape1/1  "Gravity Force Body [N]"

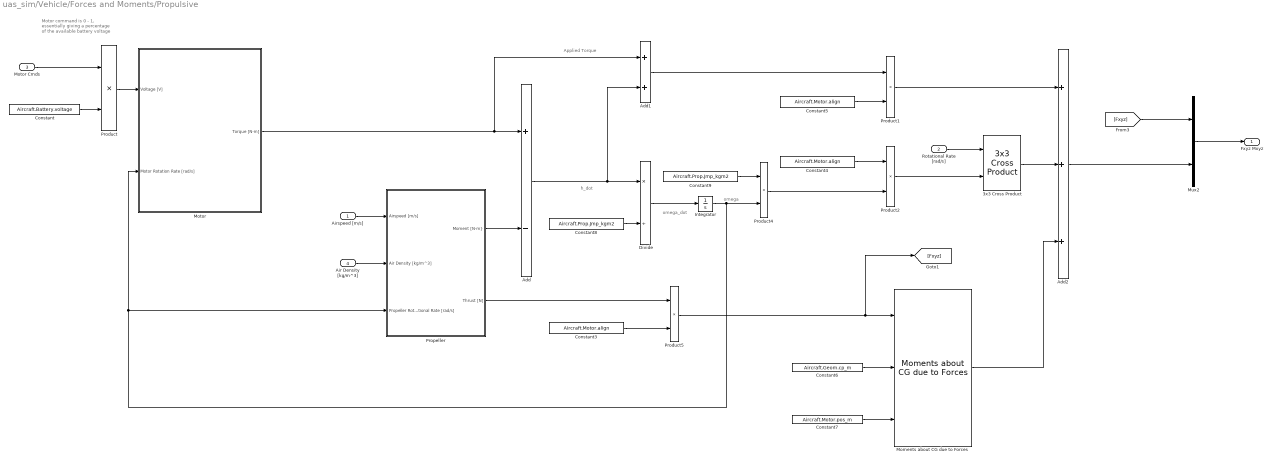
== system uas_sim/Vehicle/Forces and Moments/Propulsive ==
  note: Applied Torque
  note: omega_dot
  note: Motor command is 0 - 1,
      | essentially giving a percentage
      | of the available battery voltage
  note: h_dot
  note: omega
  Airspeed [m/s] : Inport
  Rotational Rate [rad/s] : Inport  Port=2
  Motor Cmds : Inport  Port=3
  Air Density [kg/m^3] : Inport  Port=4
  3x3 Cross Product : sharedutil/3x3 Cross Product  aMode=aMode
      settings: SourceProductBaseCode=AE,PW,MT,UV,VE,VP
  Add : Sum  Inputs=+-
  Add1 : Sum
  Add2 : Sum  Inputs=+++
  Constant : Constant  Value=Aircraft.Battery.voltage
  Constant3 : Constant  Value=Aircraft.Motor.align
  Constant4 : Constant  Value=Aircraft.Motor.align
  Constant5 : Constant  Value=Aircraft.Motor.align
  Constant6 : Constant  Value=Aircraft.Geom.cp_m
  Constant7 : Constant  Value=Aircraft.Motor.pos_m
  Constant8 : Constant  Value=Aircraft.Prop.Jmp_kgm2
  Constant9 : Constant  Value=Aircraft.Prop.Jmp_kgm2
  Divide : Product  Inputs=*/
  Integrator : Integrator  InitialCondition=InitCond.engine_speed_radps  LowerSaturationLimit=1
  Moments about CG due to Forces : aerolibbdyn/Moments about CG  due to Forces
      settings: SourceProductBaseCode=AE
  Motor : Subsystem
  Mux2 : Mux  Inputs=2
  Product{,1..2,4..5} (5 alike) : Product
  Propeller : Subsystem
  Fxyz Mxyz : Outport
  wires:
  Integrator/1 -> Product4/2, Propeller/3(Propeller Rotational Rate [rad/s]), Motor/2(Motor Rotation Rate [rad/s])
  [Fxyz] -> Mux2/1
  Constant4/1 -> Product2/1
  Motor/1(Torque [N-m]) -> Add1/1, Add/1
  Add1/1 -> Product1/1
  Product/1 -> Motor/1(Voltage [V])
  Moments about CG due to Forces/1 -> Add2/3
  Product1/1 -> Add2/1
  Add2/1 -> Mux2/2
  Constant9/1 -> Product4/1
  Propeller/2(Thrust [N]) -> Product5/1
  3x3 Cross Product/1 -> Add2/2
  Mux2/1 -> Fxyz Mxyz/1
  Constant/1 -> Product/2
  Product5/1 -> [Fxyz], Moments about CG due to Forces/1
  Constant3/1 -> Product5/2
  Divide/1 -> Integrator/1
  Add/1 -> Add1/2, Divide/1
  Propeller/1("Moment [N-m}") -> Add/2
  Constant6/1 -> Moments about CG due to Forces/2
  Rotational Rate [rad/s]/1 -> 3x3 Cross Product/1
  Air Density [kg/m^3]/1 -> Propeller/2(Air Density [kg/m^3])
  Product4/1 -> Product2/2
  Constant7/1 -> Moments about CG due to Forces/3
  Constant8/1 -> Divide/2
  Product2/1 -> 3x3 Cross Product/2
  Constant5/1 -> Product1/2
  Motor Cmds/1 -> Product/1
  Airspeed [m/s]/1 -> Propeller/1(Airspeed [m/s])

== system uas_sim/Vehicle/Vehicle Model/Norm ==
  2D Vector : Inport
  Product : Product
  Sqrt : Sqrt  SaturateOnIntegerOverflow=on
  Sum of Elements : Sum  Inputs=+
  Norm : Outport
  wires:
  2D Vector/1 -> Product/2, Product/1
  Product/1 -> Sum of Elements/1
  Sum of Elements/1 -> Sqrt/1
  Sqrt/1 -> Norm/1

== system uas_sim/Flight Management Unit/SenProc Model/Air Data/IAS ==
  note: Avoid negative values
  Differential Pressure [Pa] : Inport
  Add : Sum
  Constant : Constant  OutDataTypeStr=double
  Constant1 : Constant  Value=2/7  OutDataTypeStr=double
  Constant2 : Constant  OutDataTypeStr=double
  Divide : Product  Inputs=*/
  Multiply : Gain  Gain=5
  Pow : Math  Operator=pow  RndMeth=Zero  SaturateOnIntegerOverflow=on
  Product : Product
  Saturation : Saturate  UpperLimit=inf  LowerLimit=0
  Sqrt : Sqrt  SaturateOnIntegerOverflow=on
  Standard Sea Level Pressure [Pa] : Constant  Value=101325  OutDataTypeStr=double
  Standard Sea Level Speed of Sound [m/s] : Constant  Value=340.29  OutDataTypeStr=double
  Subtract : Sum  Inputs=+-
  IAS [m/s] : Outport
  wires:
  Differential Pressure [Pa]/1 -> Saturation/1
  Saturation/1 -> Divide/1
  Standard Sea Level Pressure [Pa]/1 -> Divide/2
  Divide/1 -> Add/1
  Constant/1 -> Add/2
  Constant1/1 -> Pow/2
  Add/1 -> Pow/1
  Pow/1 -> Subtract/1
  Constant2/1 -> Subtract/2
  Subtract/1 -> Multiply/1
  Multiply/1 -> Sqrt/1
  Sqrt/1 -> Product/1
  Product/1 -> IAS [m/s]/1
  Standard Sea Level Speed of Sound [m/s]/1 -> Product/2

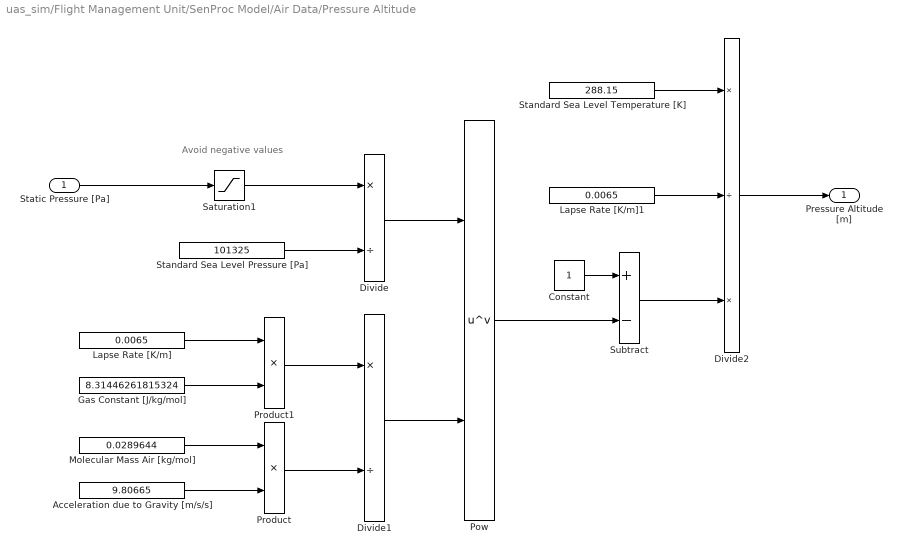
== system uas_sim/Flight Management Unit/SenProc Model/Air Data/Pressure Altitude ==
  note: Avoid negative values
  Static Pressure [Pa] : Inport
  Acceleration due to Gravity [m/s/s] : Constant  Value=9.80665  OutDataTypeStr=double
  Constant : Constant  OutDataTypeStr=double
  Divide : Product  Inputs=*/
  Divide1 : Product  Inputs=*/
  Divide2 : Product  Inputs=*/*
  Gas Constant [J/kg/mol] : Constant  Value=8.31446261815324  OutDataTypeStr=double
  Lapse Rate [K/m] : Constant  Value=0.0065  OutDataTypeStr=double
  Lapse Rate [K/m]1 : Constant  Value=0.0065  OutDataTypeStr=double
  Molecular Mass Air [kg/mol] : Constant  Value=0.0289644  OutDataTypeStr=double
  Pow : Math  Operator=pow  RndMeth=Zero  SaturateOnIntegerOverflow=on
  Product : Product
  Product1 : Product
  Saturation1 : Saturate  UpperLimit=inf  LowerLimit=0
  Standard Sea Level Pressure [Pa] : Constant  Value=101325  OutDataTypeStr=double
  Standard Sea Level Temperature [K] : Constant  Value=288.15  OutDataTypeStr=double
  Subtract : Sum  Inputs=+-
  Pressure Altitude [m] : Outport
  wires:
  Static Pressure [Pa]/1 -> Saturation1/1
  Saturation1/1 -> Divide/1
  Standard Sea Level Pressure [Pa]/1 -> Divide/2
  Divide/1 -> Pow/1
  Product1/1 -> Divide1/1
  Product/1 -> Divide1/2
  Molecular Mass Air [kg/mol]/1 -> Product/1
  Acceleration due to Gravity [m/s/s]/1 -> Product/2
  Gas Constant [J/kg/mol]/1 -> Product1/2
  Lapse Rate [K/m]/1 -> Product1/1
  Divide1/1 -> Pow/2
  Pow/1 -> Subtract/2
  Constant/1 -> Subtract/1
  Subtract/1 -> Divide2/3
  Divide2/1 -> Pressure Altitude [m]/1
  Lapse Rate [K/m]1/1 -> Divide2/2
  Standard Sea Level Temperature [K]/1 -> Divide2/1

== system uas_sim/Flight Management Unit/Sensor Models/Airdata/Differential Pressure Sensor ==
  Pressure : Inport
  Add : Sum  Inputs=+++
  Band-Limited White Noise : simulink/Sources/Band-Limited White Noise  Cov=Aircraft.Sensors.DiffPres.noise_pa  Ts=0.1  seed=[23341]
  Constant : Constant  Value=Aircraft.Sensors.DiffPres.bias_pa
  Constant1 : Constant  Value=Aircraft.Sensors.DiffPres.scale_factor
  Product : Product
  Saturation : Saturate  UpperLimit=Aircraft.Sensors.DiffPres.upper_limit_pa  LowerLimit=Aircraft.Sensors.DiffPres.lower_limit_pa
  Sensed Value : Outport
  wires:
  Constant1/1 -> Product/2
  Pressure/1 -> Product/1
  Product/1 -> Add/3
  Add/1 -> Saturation/1
  Constant/1 -> Add/2
  Band-Limited White Noise/1 -> Add/1
  Saturation/1 -> Sensed Value/1

== system uas_sim/Flight Management Unit/Sensor Models/Airdata/Static Pressure Sensor ==
  Pressure : Inport
  Add : Sum  Inputs=+++
  Band-Limited White Noise : simulink/Sources/Band-Limited White Noise  Cov=Aircraft.Sensors.StaticPres.noise_pa  Ts=0.1  seed=[23341]
  Constant : Constant  Value=Aircraft.Sensors.StaticPres.bias_pa
  Constant1 : Constant  Value=Aircraft.Sensors.StaticPres.scale_factor
  Product : Product
  Saturation : Saturate  UpperLimit=Aircraft.Sensors.StaticPres.upper_limit_pa  LowerLimit=Aircraft.Sensors.StaticPres.lower_limit_pa
  Sensed Value : Outport
  wires:
  Saturation/1 -> Sensed Value/1
  Band-Limited White Noise/1 -> Add/1
  Constant/1 -> Add/2
  Add/1 -> Saturation/1
  Product/1 -> Add/3
  Pressure/1 -> Product/1
  Constant1/1 -> Product/2

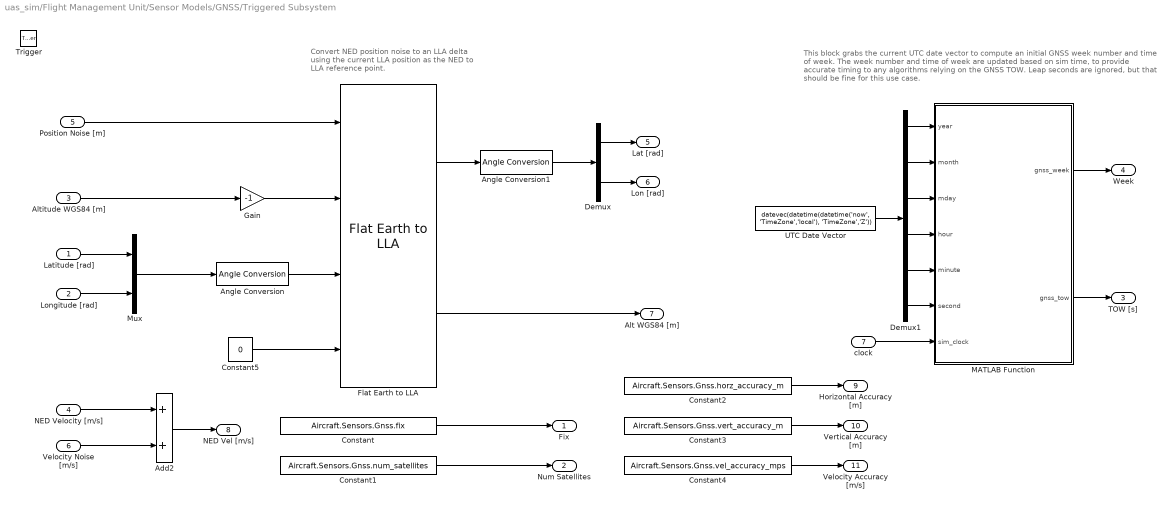
== system uas_sim/Flight Management Unit/Sensor Models/GNSS/Triggered Subsystem ==
  note: This block grabs the current UTC date vector to compute an initial GNSS week number
      | and time of week. The week number and time of week are updated based on sim time, to provide accurate timing to any algorithms relying on the GNSS TOW. Leap seconds are ignored, but that should be fine for this use case.
  note: Convert NED position noise to an LLA delta
      | using the current LLA position as the NED to
      | LLA reference point.
  Latitude [rad] : Inport
  "Longitude [rad] " : Inport  Port=2
  Altitude WGS84 [m] : Inport  Port=3
  NED Velocity [m/s] : Inport  Port=4  PortDimensions=3
  Position Noise [m] : Inport  Port=5  PortDimensions=3
  Velocity Noise [m/s] : Inport  Port=6  PortDimensions=3
  clock : Inport  Port=7
  Trigger : TriggerPort  VariantControl=Variant
  Add2 : Sum
  Angle Conversion : aerolibconvert2/Angle Conversion  IU=rad  OU=deg
  Angle Conversion1 : aerolibconvert2/Angle Conversion  IU=deg  OU=rad
  Constant : Constant  Value=Aircraft.Sensors.Gnss.fix
  Constant1 : Constant  Value=Aircraft.Sensors.Gnss.num_satellites
  Constant2 : Constant  Value=Aircraft.Sensors.Gnss.horz_accuracy_m
  Constant3 : Constant  Value=Aircraft.Sensors.Gnss.vert_accuracy_m
  Constant4 : Constant  Value=Aircraft.Sensors.Gnss.vel_accuracy_mps
  Constant5 : Constant  Value=0
  Demux : Demux  Outputs=2
  Demux1 : Demux  Outputs=6
  Flat Earth to LLA : aerolibtransform2/Flat Earth to LLA  units=Metric (MKS)  ptype=Earth (WGS84)  F=1/298.257223563  R=6378137  refPosPort=on  LL0=[0 10]  psi=0
  Gain : Gain  Gain=-1
  MATLAB Function : MATLAB Function  TreatAsAtomicUnit=on
  Mux : Mux  Inputs=2
  UTC Date Vector : Constant  Value=datevec(datetime(datetime('now', 'TimeZone','local'), 'TimeZone','Z'))  SampleTime=-1
  Fix : Outport
  Num Satellites : Outport  Port=2
  TOW [s] : Outport  Port=3
  Week : Outport  Port=4
  Lat [rad] : Outport  Port=5
  Lon [rad] : Outport  Port=6
  Alt WGS84 [m] : Outport  Port=7
  NED Vel [m/s] : Outport  Port=8
  Horizontal Accuracy [m] : Outport  Port=9
  Vertical Accuracy [m] : Outport  Port=10
  Velocity Accuracy [m/s] : Outport  Port=11
  wires:
  Constant/1 -> Fix/1
  Constant1/1 -> Num Satellites/1
  Constant2/1 -> Horizontal Accuracy [m]/1
  Constant3/1 -> Vertical Accuracy [m]/1
  Constant4/1 -> Velocity Accuracy [m/s]/1
  Position Noise [m]/1 -> Flat Earth to LLA/1
  Altitude WGS84 [m]/1 -> Gain/1
  Mux/1 -> Angle Conversion/1
  Angle Conversion/1 -> Flat Earth to LLA/3
  Constant5/1 -> Flat Earth to LLA/4
  "Longitude [rad] "/1 -> Mux/2
  Latitude [rad]/1 -> Mux/1
  Flat Earth to LLA/1 -> Angle Conversion1/1
  Angle Conversion1/1 -> Demux/1
  Demux/2 -> Lon [rad]/1
  Demux/1 -> Lat [rad]/1
  Flat Earth to LLA/2 -> Alt WGS84 [m]/1
  NED Velocity [m/s]/1 -> Add2/1
  Velocity Noise [m/s]/1 -> Add2/2
  Add2/1 -> NED Vel [m/s]/1
  Demux1/2 -> MATLAB Function/2(month)
  Demux1/6 -> MATLAB Function/6(second)
  UTC Date Vector/1 -> Demux1/1
  Demux1/1 -> MATLAB Function/1(year)
  Demux1/5 -> MATLAB Function/5(minute)
  Demux1/4 -> MATLAB Function/4(hour)
  Demux1/3 -> MATLAB Function/3(mday)
  MATLAB Function/2(gnss_tow) -> TOW [s]/1
  MATLAB Function/1(gnss_week) -> Week/1
  clock/1 -> MATLAB Function/7(sim_clock)
  Gain/1 -> Flat Earth to LLA/2
